simulink model "gm_MATE_HDLsolver_myFirstCircuit"  (R2024b)
settings: Solver=FixedStepDiscrete  StartTime=0.0  StopTime=0.05  FixedStep=6.02409638554217e-09  MaxStep=100e-6  RelTol=1e-4
PostLoadFcn:
  | Ts=1e-6; nb_sw=3; nb_lc=2;nb_r=1;nb_src=1; nb_out=3; rL=1.2;rC=100;L=1e-3; C=1e-5; LpejoSw=1e-6;h=Ts; MAX_INPUTS=16;
  | MAX_OUTPUTS=16;
  | MAX_SWITCHES=8;
  | MAX_INPUTS=16;
InitFcn:
  | Ts=1e-6; nb_sw=3; nb_lc=2;nb_r=1;nb_src=1; nb_out=3; rL=1.2;rC=100;L=1e-3; C=1e-5; LpejoSw=1e-6;h=Ts; MAX_INPUTS=16;
  | MAX_OUTPUTS=16;
  | MAX_SWITCHES=8;
  | MAX_INPUTS=16;
undefined symbols (not defined in the file or in its folder): MATE_SOC
libraries: fl_lib x31, nesl_utility x13, hdlmdlgenlib x10, simetranss x5, simulink x4, hdlsllib x3, ee_lib x2, eeGeneralControl x1
(part 8 of 8)

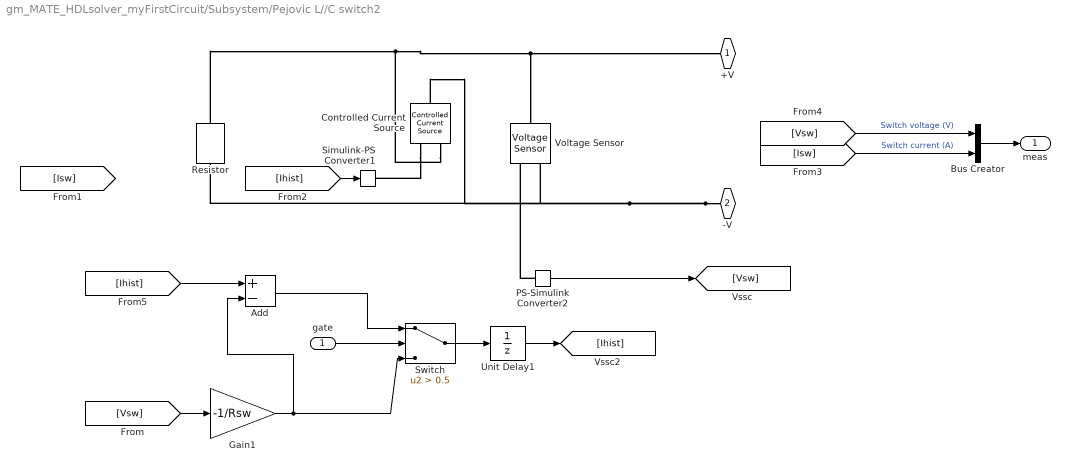
== system gm_MATE_HDLsolver_myFirstCircuit/Subsystem/Pejovic L//C switch2 ==
  gate : Inport
  Add : Sum  Inputs=+-
  Bus Creator : BusCreator  Inputs=2
  Controlled Current Source : fl_lib/Electrical/Electrical Sources/Controlled Current Source
  Gain1 : Gain  Gain=-1/Rsw
  PS-Simulink Converter2 : nesl_utility/PS-Simulink Converter  PhysicalDomain=network_engine_domain  SubClassName=ps_output  LeftPortType=input  RightPortType=output  PseudoPeriodic=off  Frequencies=[]  VectorFormat=inherit  Unit=inherit  AffineConversion=off
  Resistor : fl_lib/Electrical/Electrical Elements/Resistor  R=Rsw Ohm  i_specify=off  i_priority=None  i=0 A  i_nominal_specify=off  i_nominal_value=1  i_nominal_unit=A  v_specify=off  v_priority=None  v=0 V  v_nominal_specify=off  v_nominal_value=1  v_nominal_unit=V
  Simulink-PS Converter1 : nesl_utility/Simulink-PS Converter  PhysicalDomain=network_engine_domain  SubClassName=ps_input  LeftPortType=input  RightPortType=output  PseudoPeriodic=off  Frequencies=[]  NoiseDistribution=none  NoiseParameters=[]  Unit=1  AffineConversion=off  FilteringAndDerivatives=provide  SimscapeFilterOrder=1  InputFilterTimeConstant=0.001  UdotUserProvided=0
  Switch : Switch  Criteria=u2 > Threshold  Threshold=0.5  SaturateOnIntegerOverflow=off  InputSameDT=off
  Unit Delay1 : UnitDelay  SampleTime=-1  HasFrameUpgradeWarning=on
  Voltage Sensor : fl_lib/Electrical/Electrical Sensors/Voltage Sensor
  +V : PMIOPort  Side=Left
  -V : PMIOPort  Port=2  Side=Right
  meas : Outport
  wires:
  Bus Creator/1 -> meas/1
  [Vsw] -> Bus Creator/1  "Switch voltage (V)"
  [Isw] -> Bus Creator/2  "Switch current (A)"
  [Ihist] -> Simulink-PS Converter1/1
  Switch/1 -> Unit Delay1/1
  [Vsw] -> Gain1/1
  gate/1 -> Switch/2
  PS-Simulink Converter2/1 -> [Vsw]
  [Ihist] -> Add/1
  Gain1/1 -> Switch/3, Add/2
  Add/1 -> Switch/1
  Unit Delay1/1 -> [Ihist]
  connections:
  Resistor/LConn1 -- Controlled Current Source/RConn2 -- +V/RConn1 -- Voltage Sensor/LConn1
  Controlled Current Source/RConn1 -- Simulink-PS Converter1/RConn1
  PS-Simulink Converter2/LConn1 -- Voltage Sensor/RConn1
  -V/RConn1 -- Voltage Sensor/RConn2 -- Controlled Current Source/LConn1 -- Resistor/RConn1

== system gm_MATE_HDLsolver_myFirstCircuit/Subsystem/current measure ==
  Current Sensor2 : fl_lib/Electrical/Electrical Sensors/Current Sensor
  PS-Simulink Converter1 : nesl_utility/PS-Simulink Converter  PhysicalDomain=network_engine_domain  SubClassName=ps_output  LeftPortType=input  RightPortType=output  PseudoPeriodic=off  Frequencies=[]  VectorFormat=inherit  Unit=inherit  AffineConversion=off
  + : PMIOPort  Side=Left
  - : PMIOPort  Port=2  Side=Right
  i : Outport
  wires:
  PS-Simulink Converter1/1 -> i/1
  connections:
  Current Sensor2/RConn2 -- -/RConn1
  Current Sensor2/LConn1 -- +/RConn1
  PS-Simulink Converter1/LConn1 -- Current Sensor2/RConn1

== system gm_MATE_HDLsolver_myFirstCircuit/ForFPGA/Counter Free-Running/Increment Real World ==
  u : Inport  OutDataTypeStr=fixdt(0,4,0,'DataTypeOverride', 'Off')  SampleTime=1e-06
  FixPt Constant : Constant  DisableCoverage=on  OutDataTypeStr=fixdt(0, 4, 0)  SampleTime=-1
  FixPt Sum1 : Sum  OutDataTypeStr=fixdt(0, 4, 0)  InputSameDT=on  LockScale=on
  y : Outport  SampleTime=1e-06
  wires:
  FixPt Sum1/1 -> y/1
  u/1 -> FixPt Sum1/1
  FixPt Constant/1 -> FixPt Sum1/2

== system gm_MATE_HDLsolver_myFirstCircuit/ForFPGA/Counter Free-Running/Wrap To Zero ==
  note: U(k)
  U : Inport  OutDataTypeStr=fixdt(0,4,0,'DataTypeOverride', 'Off')  SampleTime=1e-06
  Constant : Constant  DisableCoverage=on  Value=0  OutDataTypeStr=fixdt(0, 4, 0)  SampleTime=-1
  FixPt Switch : Switch  Criteria=u2 > Threshold  Threshold=Threshold  OutDataTypeStr=fixdt(0, 4, 0)  ZeroCross=off  SaturateOnIntegerOverflow=off  InputSameDT=off
  Y : Outport  SampleTime=1e-06
  wires:
  Constant/1 -> FixPt Switch/1
  U/1 -> FixPt Switch/3, FixPt Switch/2
  FixPt Switch/1 -> Y/1

== system gm_MATE_HDLsolver_myFirstCircuit/ForFPGA/LC vectorized/Add ==
  In1 : Inport
  In2 : Inport  Port=2
  Add : Sum  Inputs=+-  OutDataTypeStr=single  SampleTime=6.02409638554217e-09
  Add_pd1 : Delay  DelayLength=6
  Out1 : Outport
  wires:
  In1/1 -> Add/1
  In2/1 -> Add/2
  Add/1 -> Add_pd1/1
  Add_pd1/1 -> Out1/1

== system gm_MATE_HDLsolver_myFirstCircuit/ForFPGA/LC vectorized/Divide ==
  In1 : Inport
  In2 : Inport  Port=2
  Divide : Product  Inputs=**  OutDataTypeStr=single  SampleTime=6.02409638554217e-09
  Divide_pd1 : Delay  DelayLength=6
  Out1 : Outport
  wires:
  In1/1 -> Divide/1
  In2/1 -> Divide/2
  Divide/1 -> Divide_pd1/1
  Divide_pd1/1 -> Out1/1

== system gm_MATE_HDLsolver_myFirstCircuit/ForFPGA/LC vectorized/Gain3_unaryminus ==
  In1 : Inport
  Gain3_unaryminus : UnaryMinus  SampleTime=6.02409638554217e-09
  Out1 : Outport
  wires:
  In1/1 -> Gain3_unaryminus/1
  Gain3_unaryminus/1 -> Out1/1

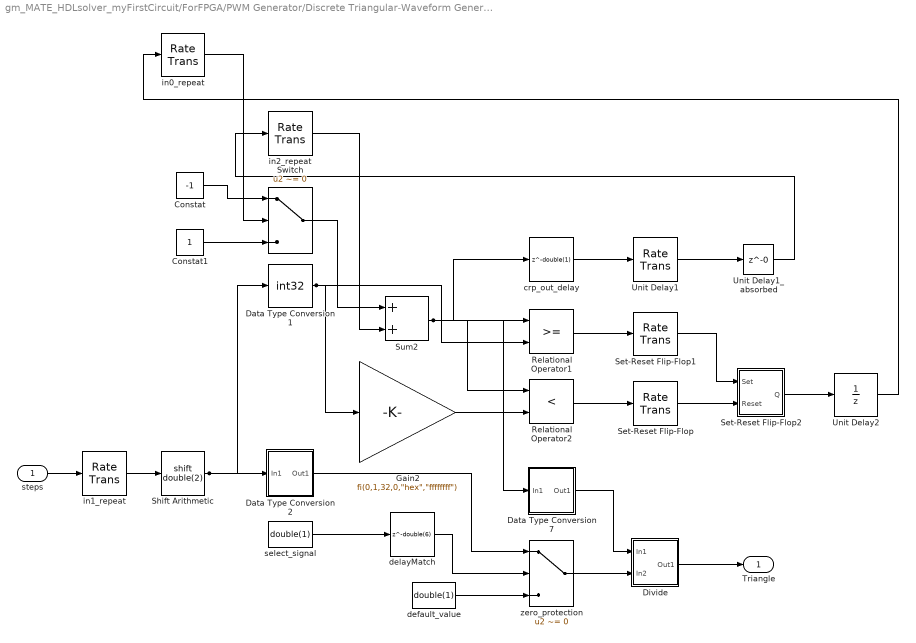
== system gm_MATE_HDLsolver_myFirstCircuit/ForFPGA/PWM Generator/Discrete Triangular-Waveform Generator ==
  steps : Inport  OutDataTypeStr=uint16  PortDimensions=1  SampleTime=1e-06
  Constat : Constant  Value=-1  OutDataTypeStr=int32  SampleTime=6.02409638554217e-09
  Constat1 : Constant  OutDataTypeStr=int32  SampleTime=6.02409638554217e-09
  Data Type Conversion1 : DataTypeConversion  OutDataTypeStr=int32  RndMeth=Nearest  SampleTime=6.02409638554217e-09  SaturateOnIntegerOverflow=off
  Data Type Conversion2 : Subsystem
      mask Display: disp('NFP\nconv');
  Data Type Conversion7 : Subsystem
      mask Display: disp('NFP\nconv');
  Divide : Subsystem
      mask Display: disp('NFP\nmul');
  Gain2 : Gain  Gain="fi(0,1,32,0,\"hex\",\"ffffffff\")"  ParamDataTypeStr=fixdt(1, 32, 0)  OutDataTypeStr=int32  SaturateOnIntegerOverflow=on  SampleTime=6.02409638554217e-09
  Relational Operator1 : RelationalOperator  OutDataTypeStr=boolean  SampleTime=6.02409638554217e-09
  Relational Operator2 : RelationalOperator  Operator=<  OutDataTypeStr=boolean  SampleTime=6.02409638554217e-09
  Set-Reset Flip-Flop : RateTransition  InitialCondition=double(0)  OutPortSampleTimeOpt=Multiple of input port sample time  OutPortSampleTimeMultiple=166
  Set-Reset Flip-Flop1 : RateTransition  InitialCondition=double(0)  OutPortSampleTimeOpt=Multiple of input port sample time  OutPortSampleTimeMultiple=166
  Set-Reset Flip-Flop2 : Subsystem  mask(Set-Reset Flip-Flop){UndefState=Set, Q0=double(0), Ts=double(1e-06)}
      mask prompts: UndefState "physmod:ee:library:comments:control:eeGeneralControl:PriorityWhenUndefinedState_MP"; Q0 "physmod:ee:library:comments:control:eeGeneralControl:InitialConditionForQState_MP"; Ts "physmod:ee:library:comments:control:eeGeneralControl:SampleTime1ForInherited_MP"
      mask help: physmod:ee:library:comments:control:eeGeneralControl:SetResetFlipFlop_MD
      mask init:
      | Q0 = double(0);
      | Ts = double(1e-06);
      | UndefState = double(2);
      | isSetWhenUndefinedState = double(1);
      | timeDomain = 'Discrete';
      mask Help: web(nesl_help(gcbh))
      mask TypeOptions UndefState: physmod:ee:library:comments:control:eeGeneralControl:Reset_PV | physmod:ee:library:comments:control:eeGeneralControl:Set_PV
      mask Display: ee.mask.drawSetResetFlipFlop;
  Shift Arithmetic : ArithShift  BitShiftNumber=double(2)  BinPtShiftNumber=double(0)
  Sum2 : Sum  OutDataTypeStr=int32  AccumDataTypeStr=int32  SaturateOnIntegerOverflow=on  SampleTime=6.02409638554217e-09
  Switch : Switch  Criteria=u2 ~= 0  Threshold=double(0)  OutDataTypeStr=int32  SampleTime=6.02409638554217e-09  InputSameDT=off
  Unit Delay1 : RateTransition  InitialCondition=double(0)  OutPortSampleTimeOpt=Multiple of input port sample time  OutPortSampleTimeMultiple=166
  Unit Delay1_absorbed : Delay  DelayLength=0
  Unit Delay2 : UnitDelay  SampleTime=1e-06
  crp_out_delay : Delay  DelayLength=double(1)  InitialCondition=0  SampleTime=6.02409638554217e-09
  default_value : Constant  Value=double(1)  OutDataTypeStr=single  SampleTime=6.02409638554217e-09
  delayMatch : Delay  DelayLength=double(6)  InitialCondition=0  SampleTime=6.02409638554217e-09
  in0_repeat : RateTransition  Integrity=off  Deterministic=off  OutPortSampleTimeOpt=Multiple of input port sample time  OutPortSampleTimeMultiple=1/166
  in1_repeat : RateTransition  Integrity=off  Deterministic=off  OutPortSampleTimeOpt=Multiple of input port sample time  OutPortSampleTimeMultiple=1/166
  in2_repeat : RateTransition  Integrity=off  Deterministic=off  OutPortSampleTimeOpt=Multiple of input port sample time  OutPortSampleTimeMultiple=1/166
  select_signal : Constant  Value=double(1)  OutDataTypeStr=boolean  SampleTime=6.02409638554217e-09
  zero_protection : Switch  Criteria=u2 ~= 0  Threshold=double(0)  OutDataTypeStr=single  SampleTime=6.02409638554217e-09  SaturateOnIntegerOverflow=off  InputSameDT=off
  Triangle : Outport  SampleTime=6.02409638554217e-09  InitialOutput=0  VectorParamsAs1DForOutWhenUnconnected=off
  wires:
  steps/1 -> in1_repeat/1
  select_signal/1 -> delayMatch/1
  Constat/1 -> Switch/1
  in1_repeat/1 -> Shift Arithmetic/1
  in0_repeat/1 -> Switch/2
  Constat1/1 -> Switch/3
  Switch/1 -> Sum2/1
  in2_repeat/1 -> Sum2/2
  Shift Arithmetic/1 -> Data Type Conversion2/1(In1), Data Type Conversion1/1
  Data Type Conversion1/1 -> Relational Operator1/2, Gain2/1
  Data Type Conversion2/1(Out1) -> zero_protection/1
  crp_out_delay/1 -> Unit Delay1/1
  Sum2/1 -> Data Type Conversion7/1(In1), Relational Operator1/1, Relational Operator2/1, crp_out_delay/1
  Gain2/1 -> Relational Operator2/2
  delayMatch/1 -> zero_protection/2
  zero_protection/1 -> Divide/2(In2)
  default_value/1 -> zero_protection/3
  Relational Operator1/1 -> Set-Reset Flip-Flop1/1
  Relational Operator2/1 -> Set-Reset Flip-Flop/1
  Data Type Conversion7/1(Out1) -> Divide/1(In1)
  Unit Delay1/1 -> Unit Delay1_absorbed/1
  Set-Reset Flip-Flop1/1 -> Set-Reset Flip-Flop2/1(Set)
  Set-Reset Flip-Flop/1 -> Set-Reset Flip-Flop2/2(Reset)
  Divide/1(Out1) -> Triangle/1
  Unit Delay1_absorbed/1 -> in2_repeat/1
  Set-Reset Flip-Flop2/1(Q) -> Unit Delay2/1
  Unit Delay2/1 -> in0_repeat/1

== system gm_MATE_HDLsolver_myFirstCircuit/ForFPGA/PWM Generator/Relational Operator ==
  In1 : Inport
  In2 : Inport  Port=2
  Relational Operator : RelationalOperator  OutDataTypeStr=boolean  SampleTime=6.02409638554217e-09
  Relational Operator_pd1 : Delay  DelayLength=1
  Out1 : Outport
  wires:
  In1/1 -> Relational Operator/1
  In2/1 -> Relational Operator/2
  Relational Operator/1 -> Relational Operator_pd1/1
  Relational Operator_pd1/1 -> Out1/1

== system gm_MATE_HDLsolver_myFirstCircuit/ForFPGA/PWM Generator/Discrete Triangular-Waveform Generator/Data Type Conversion2 ==
  In1 : Inport
  Data Type Conversion2 : DataTypeConversion  OutDataTypeStr=single  RndMeth=Nearest  SampleTime=6.02409638554217e-09  SaturateOnIntegerOverflow=off
  Data Type Conversion2_pd1 : Delay  DelayLength=6
  Out1 : Outport
  wires:
  In1/1 -> Data Type Conversion2/1
  Data Type Conversion2/1 -> Data Type Conversion2_pd1/1
  Data Type Conversion2_pd1/1 -> Out1/1

== system gm_MATE_HDLsolver_myFirstCircuit/ForFPGA/PWM Generator/Discrete Triangular-Waveform Generator/Data Type Conversion7 ==
  In1 : Inport
  Data Type Conversion7 : DataTypeConversion  OutDataTypeStr=single  RndMeth=Nearest  SampleTime=6.02409638554217e-09  SaturateOnIntegerOverflow=off
  Data Type Conversion7_pd1 : Delay  DelayLength=6
  Out1 : Outport
  wires:
  In1/1 -> Data Type Conversion7/1
  Data Type Conversion7/1 -> Data Type Conversion7_pd1/1
  Data Type Conversion7_pd1/1 -> Out1/1

== system gm_MATE_HDLsolver_myFirstCircuit/ForFPGA/PWM Generator/Discrete Triangular-Waveform Generator/Divide ==
  In1 : Inport
  In2 : Inport  Port=2
  Divide : Product  Inputs=*/  OutDataTypeStr=single  SampleTime=6.02409638554217e-09
  Divide_pd1 : Delay  DelayLength=17
  Out1 : Outport
  wires:
  In1/1 -> Divide/1
  In2/1 -> Divide/2
  Divide/1 -> Divide_pd1/1
  Divide_pd1/1 -> Out1/1

== system gm_MATE_HDLsolver_myFirstCircuit/ForFPGA/PWM Generator/Discrete Triangular-Waveform Generator/Set-Reset Flip-Flop2 ==
  Set : Inport  OutDataTypeStr=boolean  SampleTime=1e-06
  Reset : Inport  Port=2  OutDataTypeStr=boolean  SampleTime=1e-06
  Discrete : Subsystem
  Q : Outport  SampleTime=1e-06
  wires:
  Discrete/1(Q) -> Q/1
  Set/1 -> Discrete/1(Set)
  Reset/1 -> Discrete/2(Reset)

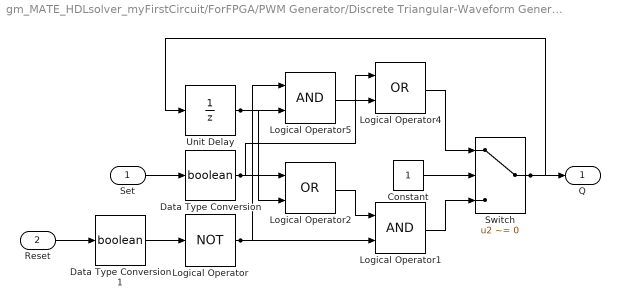
== system gm_MATE_HDLsolver_myFirstCircuit/ForFPGA/PWM Generator/Discrete Triangular-Waveform Generator/Set-Reset Flip-Flop2/Discrete ==
  Set : Inport  OutDataTypeStr=boolean  PortDimensions=1  SampleTime=1e-06
  Reset : Inport  Port=2  OutDataTypeStr=boolean  PortDimensions=1  SampleTime=1e-06
  Constant : Constant  OutDataTypeStr=boolean  SampleTime=1e-06
  Data Type Conversion : DataTypeConversion  OutDataTypeStr=boolean
  Data Type Conversion1 : DataTypeConversion  OutDataTypeStr=boolean
  Logical Operator : Logic  Operator=NOT  Inputs=1  AllPortsSameDT=off  OutDataTypeStr=boolean  SampleTime=1e-06
  Logical Operator1 : Logic  AllPortsSameDT=off  OutDataTypeStr=boolean  SampleTime=1e-06
  Logical Operator2 : Logic  Operator=OR  AllPortsSameDT=off  OutDataTypeStr=boolean  SampleTime=1e-06
  Logical Operator4 : Logic  Operator=OR  AllPortsSameDT=off  OutDataTypeStr=boolean  SampleTime=1e-06
  Logical Operator5 : Logic  AllPortsSameDT=off  OutDataTypeStr=boolean  SampleTime=1e-06
  Switch : Switch  Criteria=u2 ~= 0  Threshold=double(0)  OutDataTypeStr=boolean  SampleTime=1e-06  SaturateOnIntegerOverflow=off  InputSameDT=off
  Unit Delay : UnitDelay  SampleTime=1e-06
  Q : Outport  SampleTime=1e-06  VectorParamsAs1DForOutWhenUnconnected=off
  wires:
  Data Type Conversion1/1 -> Logical Operator/1
  Set/1 -> Data Type Conversion/1
  Logical Operator4/1 -> Switch/1
  Reset/1 -> Data Type Conversion1/1
  Logical Operator/1 -> Logical Operator1/2, Logical Operator5/1
  Constant/1 -> Switch/2
  Unit Delay/1 -> Logical Operator2/2, Logical Operator5/2
  Logical Operator5/1 -> Logical Operator4/2
  Data Type Conversion/1 -> Logical Operator4/1, Logical Operator2/1
  Logical Operator2/1 -> Logical Operator1/1
  Logical Operator1/1 -> Switch/3
  Switch/1 -> Unit Delay/1, Q/1
